simulink model "VehicleECU"  (R2018b)
settings: configuration reference "Active" (kept outside this file)
undefined symbols (not defined in the file): TUMHealthStatus, TUMStrategyState
settings Model: DataDictionary=VehicleECU.sldd  sg_rtwmakecfg_data=_sglibc_  ExplicitPartitioning=on  Creator=wischnewski  LastModifiedBy=ge34qer

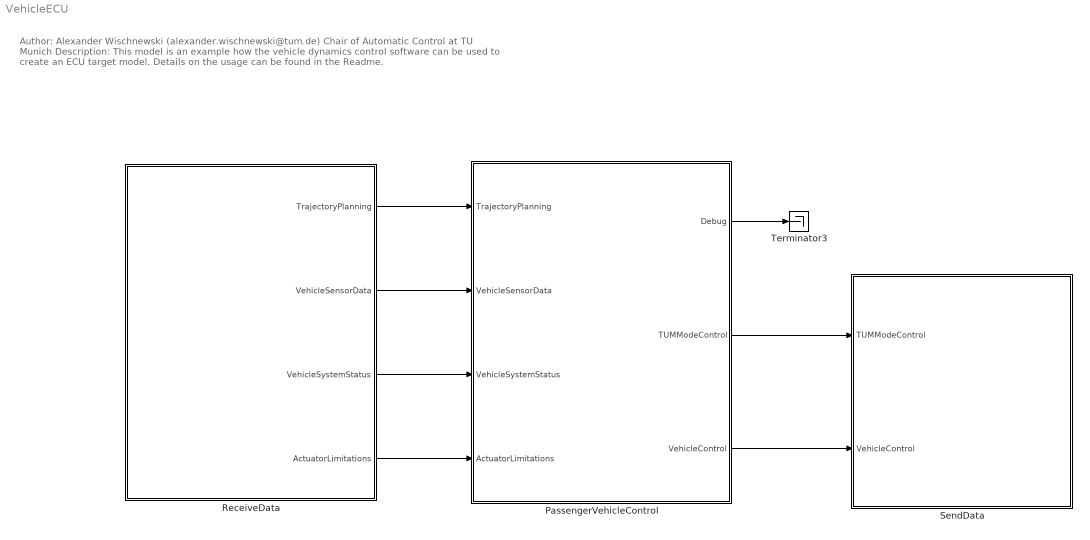
== system VehicleECU ==
  note: Author: Alexander Wischnewski (alexander.wischnewski@tum.de)
      | Chair of Automatic Control at TU Munich
      |
      | Description: This model is an example how the vehicle dynamics control software can be used to create an ECU target model. Details
      | on the usage can be found in the Readme.
  PassengerVehicleControl : Subsystem
  ReceiveData : Subsystem
  SendData : Subsystem
  Terminator3 : Terminator
  wires:
  ReceiveData/1(TrajectoryPlanning) -> PassengerVehicleControl/1(TrajectoryPlanning)
  ReceiveData/2(VehicleSensorData) -> PassengerVehicleControl/2(VehicleSensorData)
  ReceiveData/3(VehicleSystemStatus) -> PassengerVehicleControl/3(VehicleSystemStatus)
  ReceiveData/4(ActuatorLimitations) -> PassengerVehicleControl/4(ActuatorLimitations)
  PassengerVehicleControl/3(VehicleControl) -> SendData/2(VehicleControl)
  PassengerVehicleControl/2(TUMModeControl) -> SendData/1(TUMModeControl)
  PassengerVehicleControl/1(Debug) -> Terminator3/1

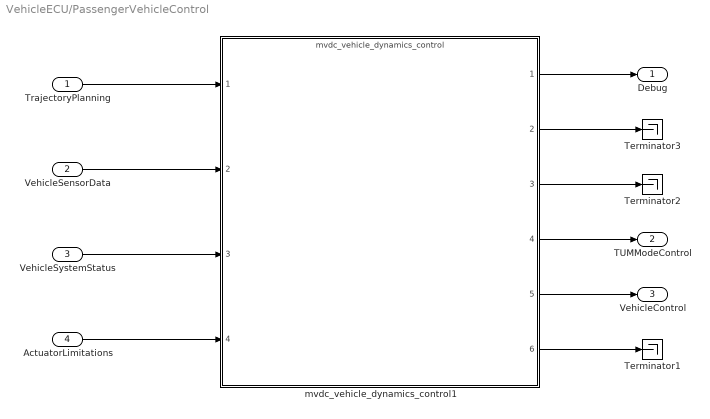
== system VehicleECU/PassengerVehicleControl ==
  TrajectoryPlanning : Inport
  VehicleSensorData : Inport  Port=2
  VehicleSystemStatus : Inport  Port=3
  ActuatorLimitations : Inport  Port=4
  Terminator1 : Terminator
  Terminator2 : Terminator
  Terminator3 : Terminator
  mvdc_vehicle_dynamics_control1 : ModelReference  ModelNameDialog=mvdc_vehicle_dynamics_control  SimulationMode=Normal  ModelReferenceVersion=1.757
  Debug : Outport
  TUMModeControl : Outport  Port=2
  VehicleControl : Outport  Port=3
  wires:
  VehicleSystemStatus/1 -> mvdc_vehicle_dynamics_control1/3
  ActuatorLimitations/1 -> mvdc_vehicle_dynamics_control1/4
  VehicleSensorData/1 -> mvdc_vehicle_dynamics_control1/2
  TrajectoryPlanning/1 -> mvdc_vehicle_dynamics_control1/1
  mvdc_vehicle_dynamics_control1/6 -> Terminator1/1
  mvdc_vehicle_dynamics_control1/3 -> Terminator2/1
  mvdc_vehicle_dynamics_control1/2 -> Terminator3/1
  mvdc_vehicle_dynamics_control1/5 -> VehicleControl/1
  mvdc_vehicle_dynamics_control1/4 -> TUMModeControl/1
  mvdc_vehicle_dynamics_control1/1 -> Debug/1

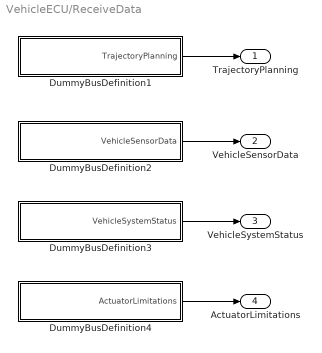
== system VehicleECU/ReceiveData ==
  DummyBusDefinition1 : Subsystem
  DummyBusDefinition2 : Subsystem
  DummyBusDefinition3 : Subsystem
  DummyBusDefinition4 : Subsystem
  TrajectoryPlanning : Outport
  VehicleSensorData : Outport  Port=2
  VehicleSystemStatus : Outport  Port=3
  ActuatorLimitations : Outport  Port=4
  wires:
  DummyBusDefinition4/1(ActuatorLimitations) -> ActuatorLimitations/1
  DummyBusDefinition3/1(VehicleSystemStatus) -> VehicleSystemStatus/1
  DummyBusDefinition2/1(VehicleSensorData) -> VehicleSensorData/1
  DummyBusDefinition1/1(TrajectoryPlanning) -> TrajectoryPlanning/1

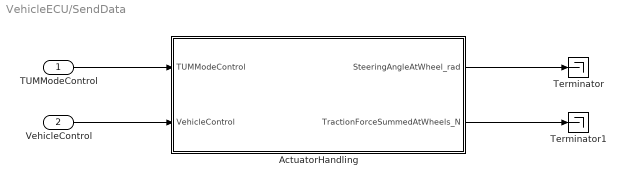
== system VehicleECU/SendData ==
  TUMModeControl : Inport  OutDataTypeStr=Bus: TUMModeControl
  VehicleControl : Inport  Port=2  OutDataTypeStr=Bus: VehicleControl
  ActuatorHandling : Subsystem
  Terminator : Terminator
  Terminator1 : Terminator
  wires:
  TUMModeControl/1 -> ActuatorHandling/1(TUMModeControl)
  VehicleControl/1 -> ActuatorHandling/2(VehicleControl)
  ActuatorHandling/1(SteeringAngleAtWheel_rad) -> Terminator/1
  ActuatorHandling/2(TractionForceSummedAtWheels_N) -> Terminator1/1

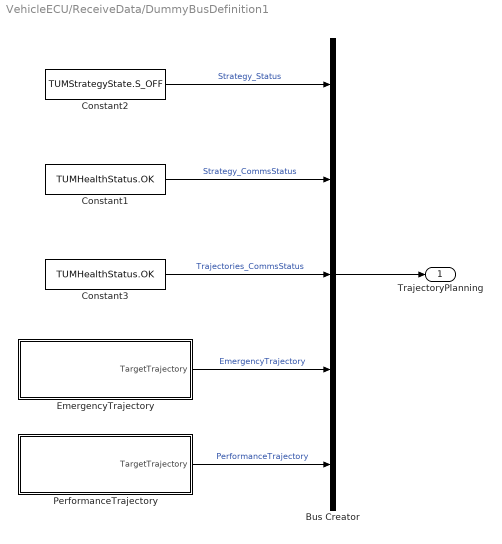
== system VehicleECU/ReceiveData/DummyBusDefinition1 ==
  Bus Creator : BusCreator  Inputs=5  OutDataTypeStr=Bus: TrajectoryPlanning
      settings: InheritFromInputs=off
  Constant1 : Constant  Value=TUMHealthStatus.OK
  Constant2 : Constant  Value=TUMStrategyState.S_OFF
  Constant3 : Constant  Value=TUMHealthStatus.OK
  EmergencyTrajectory : Subsystem  Priority=1000
  PerformanceTrajectory : Subsystem  Priority=1000
  TrajectoryPlanning : Outport
  wires:
  EmergencyTrajectory/1(TargetTrajectory) -> Bus Creator/4  "EmergencyTrajectory"
  Constant2/1 -> Bus Creator/1  "Strategy_Status"
  Constant1/1 -> Bus Creator/2  "Strategy_CommsStatus"
  Bus Creator/1 -> TrajectoryPlanning/1
  Constant3/1 -> Bus Creator/3  "Trajectories_CommsStatus"
  PerformanceTrajectory/1(TargetTrajectory) -> Bus Creator/5  "PerformanceTrajectory"

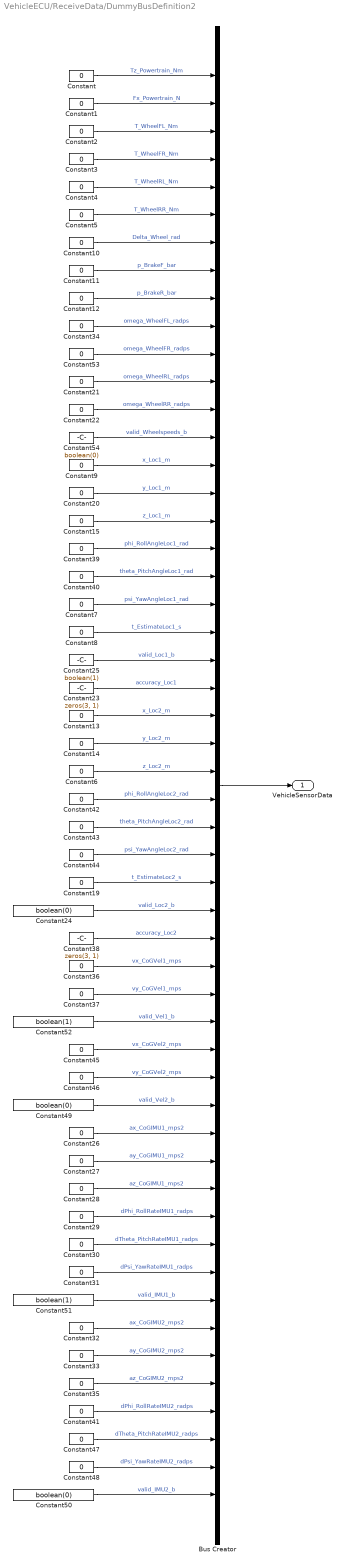
== system VehicleECU/ReceiveData/DummyBusDefinition2 ==
  Bus Creator : BusCreator  Inputs=52
  Constant{,1..15,19..22,26..37,39..48,53} (43 alike) : Constant  Value=0
  Constant23 : Constant  Value=zeros(3, 1)
  Constant{24,49..50,54} (4 alike) : Constant  Value=boolean(0)
  Constant25 : Constant  Value=boolean(1)
  Constant38 : Constant  Value=zeros(3, 1)
  Constant51 : Constant  Value=boolean(1)
  Constant52 : Constant  Value=boolean(1)
  VehicleSensorData : Outport
  wires:
  Constant1/1 -> Bus Creator/2  "Fx_Powertrain_N"
  Constant27/1 -> Bus Creator/40  "ay_CoGIMU1_mps2"
  Constant53/1 -> Bus Creator/11  "omega_WheelFR_radps"
  Constant9/1 -> Bus Creator/15  "x_Loc1_m"
  Constant30/1 -> Bus Creator/43  "dTheta_PitchRateIMU1_radps"
  Constant13/1 -> Bus Creator/24  "x_Loc2_m"
  Constant15/1 -> Bus Creator/17  "z_Loc1_m"
  Constant11/1 -> Bus Creator/8  "p_BrakeF_bar"
  Constant21/1 -> Bus Creator/12  "omega_WheelRL_radps"
  Constant5/1 -> Bus Creator/6  "T_WheelRR_Nm"
  Constant2/1 -> Bus Creator/3  "T_WheelFL_Nm"
  Bus Creator/1 -> VehicleSensorData/1
  Constant4/1 -> Bus Creator/5  "T_WheelRL_Nm"
  Constant35/1 -> Bus Creator/48  "az_CoGIMU2_mps2"
  Constant44/1 -> Bus Creator/29  "psi_YawAngleLoc2_rad"
  Constant28/1 -> Bus Creator/41  "az_CoGIMU1_mps2"
  Constant10/1 -> Bus Creator/7  "Delta_Wheel_rad"
  Constant38/1 -> Bus Creator/32  "accuracy_Loc2"
  Constant47/1 -> Bus Creator/50  "dTheta_PitchRateIMU2_radps"
  Constant45/1 -> Bus Creator/36  "vx_CoGVel2_mps"
  Constant25/1 -> Bus Creator/22  "valid_Loc1_b"
  Constant52/1 -> Bus Creator/35  "valid_Vel1_b"
  Constant22/1 -> Bus Creator/13  "omega_WheelRR_radps"
  Constant37/1 -> Bus Creator/34  "vy_CoGVel1_mps"
  Constant26/1 -> Bus Creator/39  "ax_CoGIMU1_mps2"
  Constant51/1 -> Bus Creator/45  "valid_IMU1_b"
  Constant33/1 -> Bus Creator/47  "ay_CoGIMU2_mps2"
  Constant29/1 -> Bus Creator/42  "dPhi_RollRateIMU1_radps"
  Constant20/1 -> Bus Creator/16  "y_Loc1_m"
  Constant31/1 -> Bus Creator/44  "dPsi_YawRateIMU1_radps"
  Constant8/1 -> Bus Creator/21  "t_EstimateLoc1_s"
  Constant46/1 -> Bus Creator/37  "vy_CoGVel2_mps"
  Constant40/1 -> Bus Creator/19  "theta_PitchAngleLoc1_rad"
  Constant48/1 -> Bus Creator/51  "dPsi_YawRateIMU2_radps"
  Constant36/1 -> Bus Creator/33  "vx_CoGVel1_mps"
  Constant6/1 -> Bus Creator/26  "z_Loc2_m"
  Constant41/1 -> Bus Creator/49  "dPhi_RollRateIMU2_radps"
  Constant42/1 -> Bus Creator/27  "phi_RollAngleLoc2_rad"
  Constant50/1 -> Bus Creator/52  "valid_IMU2_b"
  Constant12/1 -> Bus Creator/9  "p_BrakeR_bar"
  Constant32/1 -> Bus Creator/46  "ax_CoGIMU2_mps2"
  Constant7/1 -> Bus Creator/20  "psi_YawAngleLoc1_rad"
  Constant24/1 -> Bus Creator/31  "valid_Loc2_b"
  Constant34/1 -> Bus Creator/10  "omega_WheelFL_radps"
  Constant39/1 -> Bus Creator/18  "phi_RollAngleLoc1_rad"
  Constant/1 -> Bus Creator/1  "Tz_Powertrain_Nm"
  Constant3/1 -> Bus Creator/4  "T_WheelFR_Nm"
  Constant43/1 -> Bus Creator/28  "theta_PitchAngleLoc2_rad"
  Constant19/1 -> Bus Creator/30  "t_EstimateLoc2_s"
  Constant49/1 -> Bus Creator/38  "valid_Vel2_b"
  Constant14/1 -> Bus Creator/25  "y_Loc2_m"
  Constant23/1 -> Bus Creator/23  "accuracy_Loc1"
  Constant54/1 -> Bus Creator/14  "valid_Wheelspeeds_b"

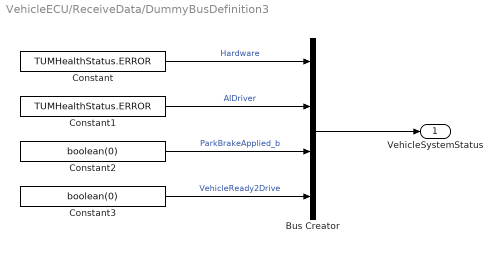
== system VehicleECU/ReceiveData/DummyBusDefinition3 ==
  Bus Creator : BusCreator  Inputs=4
  Constant : Constant  Value=TUMHealthStatus.ERROR
  Constant1 : Constant  Value=TUMHealthStatus.ERROR
  Constant2 : Constant  Value=boolean(0)
  Constant3 : Constant  Value=boolean(0)
  VehicleSystemStatus : Outport
  wires:
  Bus Creator/1 -> VehicleSystemStatus/1
  Constant/1 -> Bus Creator/1  "Hardware"
  Constant1/1 -> Bus Creator/2  "AIDriver"
  Constant2/1 -> Bus Creator/3  "ParkBrakeApplied_b"
  Constant3/1 -> Bus Creator/4  "VehicleReady2Drive"

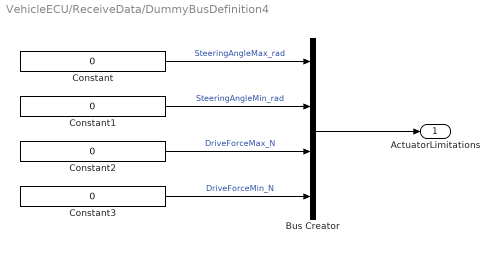
== system VehicleECU/ReceiveData/DummyBusDefinition4 ==
  Bus Creator : BusCreator  Inputs=4
  Constant{,1..3} (4 alike) : Constant  Value=0
  ActuatorLimitations : Outport
  wires:
  Bus Creator/1 -> ActuatorLimitations/1
  Constant/1 -> Bus Creator/1  "SteeringAngleMax_rad"
  Constant1/1 -> Bus Creator/2  "SteeringAngleMin_rad"
  Constant2/1 -> Bus Creator/3  "DriveForceMax_N"
  Constant3/1 -> Bus Creator/4  "DriveForceMin_N"

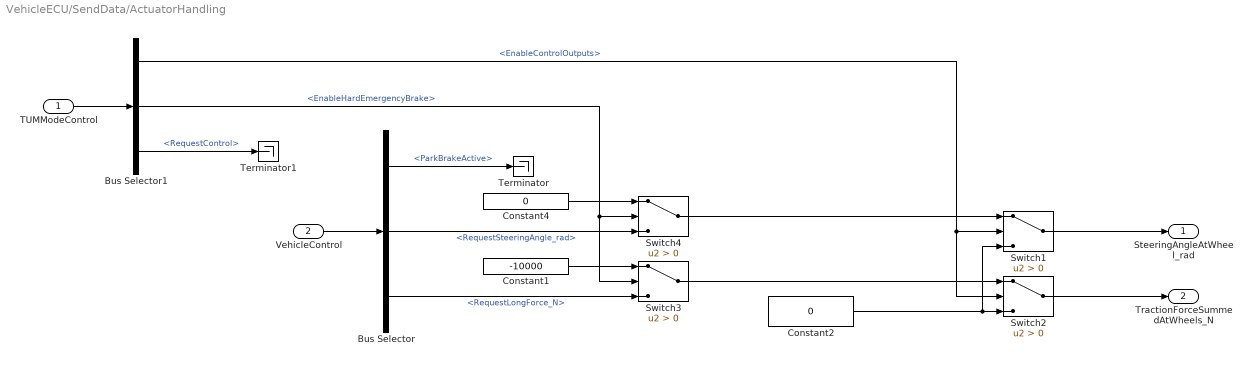
== system VehicleECU/SendData/ActuatorHandling ==
  TUMModeControl : Inport  OutDataTypeStr=Bus: TUMModeControl
  VehicleControl : Inport  Port=2  OutDataTypeStr=Bus: VehicleControl
  Bus Selector : BusSelector  OutputSignals=ParkBrakeActive,RequestSteeringAngle_rad,RequestLongForce_N
  Bus Selector1 : BusSelector  OutputSignals=EnableControlOutputs,EnableHardEmergencyBrake,RequestControl
  Constant1 : Constant  Value=-10000
  Constant2 : Constant  Value=0
  Constant4 : Constant  Value=0
  Switch{1..4} (4 alike) : Switch  Criteria=u2 > Threshold
  Terminator : Terminator
  Terminator1 : Terminator
  SteeringAngleAtWheel_rad : Outport
  TractionForceSummedAtWheels_N : Outport  Port=2
  wires:
  Bus Selector1/1 -> Switch2/2, Switch1/2  "<EnableControlOutputs>"
  TUMModeControl/1 -> Bus Selector1/1
  Bus Selector/3 -> Switch3/3  "<RequestLongForce_N>"
  Constant2/1 -> Switch1/3, Switch2/3
  VehicleControl/1 -> Bus Selector/1
  Bus Selector/2 -> Switch4/3  "<RequestSteeringAngle_rad>"
  Constant4/1 -> Switch4/1
  Constant1/1 -> Switch3/1
  Bus Selector1/2 -> Switch3/2, Switch4/2  "<EnableHardEmergencyBrake>"
  Bus Selector/1 -> Terminator/1  "<ParkBrakeActive>"
  Bus Selector1/3 -> Terminator1/1  "<RequestControl>"
  Switch4/1 -> Switch1/1
  Switch3/1 -> Switch2/1
  Switch1/1 -> SteeringAngleAtWheel_rad/1
  Switch2/1 -> TractionForceSummedAtWheels_N/1

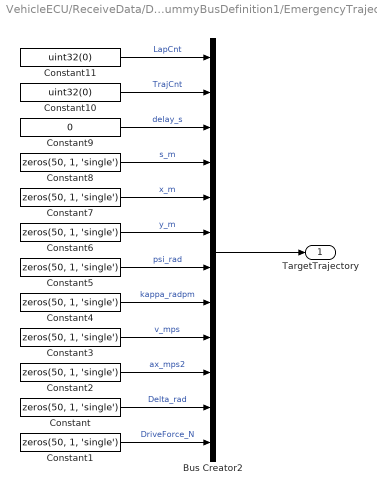
== system VehicleECU/ReceiveData/DummyBusDefinition1/EmergencyTrajectory ==
  Bus Creator2 : BusCreator  Inputs=12  OutDataTypeStr=Bus: Trajectory
      settings: InheritFromInputs=off
  Constant{,1..8} (9 alike) : Constant  Value=zeros(50, 1, 'single')
  Constant10 : Constant  Value=uint32(0)
  Constant11 : Constant  Value=uint32(0)
  Constant9 : Constant  Value=0
  TargetTrajectory : Outport  OutDataTypeStr=Bus: Trajectory
  wires:
  Constant8/1 -> Bus Creator2/4  "s_m"
  Constant7/1 -> Bus Creator2/5  "x_m"
  Constant6/1 -> Bus Creator2/6  "y_m"
  Constant5/1 -> Bus Creator2/7  "psi_rad"
  Constant4/1 -> Bus Creator2/8  "kappa_radpm"
  Constant3/1 -> Bus Creator2/9  "v_mps"
  Constant2/1 -> Bus Creator2/10  "ax_mps2"
  Constant11/1 -> Bus Creator2/1  "LapCnt"
  Constant10/1 -> Bus Creator2/2  "TrajCnt"
  Bus Creator2/1 -> TargetTrajectory/1
  Constant9/1 -> Bus Creator2/3  "delay_s"
  Constant/1 -> Bus Creator2/11  "Delta_rad"
  Constant1/1 -> Bus Creator2/12  "DriveForce_N"

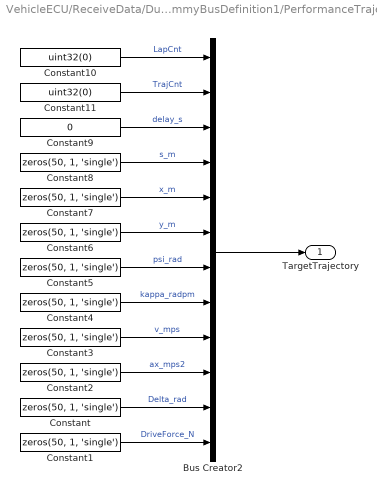
== system VehicleECU/ReceiveData/DummyBusDefinition1/PerformanceTrajectory ==
  Bus Creator2 : BusCreator  Inputs=12  OutDataTypeStr=Bus: Trajectory
      settings: InheritFromInputs=off
  Constant{,1..8} (9 alike) : Constant  Value=zeros(50, 1, 'single')
  Constant10 : Constant  Value=uint32(0)
  Constant11 : Constant  Value=uint32(0)
  Constant9 : Constant  Value=0
  TargetTrajectory : Outport  OutDataTypeStr=Bus: Trajectory
  wires:
  Constant8/1 -> Bus Creator2/4  "s_m"
  Constant7/1 -> Bus Creator2/5  "x_m"
  Constant6/1 -> Bus Creator2/6  "y_m"
  Constant5/1 -> Bus Creator2/7  "psi_rad"
  Constant4/1 -> Bus Creator2/8  "kappa_radpm"
  Constant3/1 -> Bus Creator2/9  "v_mps"
  Constant2/1 -> Bus Creator2/10  "ax_mps2"
  Constant10/1 -> Bus Creator2/1  "LapCnt"
  Constant11/1 -> Bus Creator2/2  "TrajCnt"
  Bus Creator2/1 -> TargetTrajectory/1
  Constant9/1 -> Bus Creator2/3  "delay_s"
  Constant/1 -> Bus Creator2/11  "Delta_rad"
  Constant1/1 -> Bus Creator2/12  "DriveForce_N"
